simulink model "gm_ZynqBF_2tx_fpga"  (R2018b)
settings: Solver=FixedStepDiscrete  StartTime=0.0  StopTime=10.0  FixedStep=(1/420e3)/128  RelTol=1e-3
undefined symbols (not defined in the file or in its folder): a, b, c
libraries: hdlsllib x873, simulink x349
(part 40 of 40)

== matlab function gm_ZynqBF_2tx_fpga/channel_estimator/peakdetect_ch1/correlator1/rx_ram_q_instance17/get_bit/get_bit ==
  data: u input; y output; ind input
function y = fcn(u,ind)
%#codegen

y = logical(bitget(u,ind));

== matlab function gm_ZynqBF_2tx_fpga/channel_estimator/peakdetect_ch1/correlator1/rx_ram_q_instance18/get_bit/get_bit ==
  data: u input; y output; ind input
function y = fcn(u,ind)
%#codegen

y = logical(bitget(u,ind));

== matlab function gm_ZynqBF_2tx_fpga/channel_estimator/peakdetect_ch1/correlator1/rx_ram_q_instance19/get_bit/get_bit ==
  data: u input; y output; ind input
function y = fcn(u,ind)
%#codegen

y = logical(bitget(u,ind));

== matlab function gm_ZynqBF_2tx_fpga/channel_estimator/peakdetect_ch1/correlator1/rx_ram_q_instance20/get_bit/get_bit ==
  data: u input; y output; ind input
function y = fcn(u,ind)
%#codegen

y = logical(bitget(u,ind));

== matlab function gm_ZynqBF_2tx_fpga/channel_estimator/peakdetect_ch1/correlator1/rx_ram_q_instance21/get_bit/get_bit ==
  data: u input; y output; ind input
function y = fcn(u,ind)
%#codegen

y = logical(bitget(u,ind));

== matlab function gm_ZynqBF_2tx_fpga/channel_estimator/peakdetect_ch1/correlator1/rx_ram_q_instance22/get_bit/get_bit ==
  data: u input; y output; ind input
function y = fcn(u,ind)
%#codegen

y = logical(bitget(u,ind));

== matlab function gm_ZynqBF_2tx_fpga/channel_estimator/peakdetect_ch1/correlator1/rx_ram_q_instance23/get_bit/get_bit ==
  data: u input; y output; ind input
function y = fcn(u,ind)
%#codegen

y = logical(bitget(u,ind));

== matlab function gm_ZynqBF_2tx_fpga/channel_estimator/peakdetect_ch1/correlator1/rx_ram_q_instance24/get_bit/get_bit ==
  data: u input; y output; ind input
function y = fcn(u,ind)
%#codegen

y = logical(bitget(u,ind));

== matlab function gm_ZynqBF_2tx_fpga/channel_estimator/peakdetect_ch1/correlator1/rx_ram_q_instance25/get_bit/get_bit ==
  data: u input; y output; ind input
function y = fcn(u,ind)
%#codegen

y = logical(bitget(u,ind));

== matlab function gm_ZynqBF_2tx_fpga/channel_estimator/peakdetect_ch1/correlator1/rx_ram_q_instance26/get_bit/get_bit ==
  data: u input; y output; ind input
function y = fcn(u,ind)
%#codegen

y = logical(bitget(u,ind));

== matlab function gm_ZynqBF_2tx_fpga/channel_estimator/peakdetect_ch1/correlator1/rx_ram_q_instance27/get_bit/get_bit ==
  data: u input; y output; ind input
function y = fcn(u,ind)
%#codegen

y = logical(bitget(u,ind));

== matlab function gm_ZynqBF_2tx_fpga/channel_estimator/peakdetect_ch1/correlator1/rx_ram_q_instance28/get_bit/get_bit ==
  data: u input; y output; ind input
function y = fcn(u,ind)
%#codegen

y = logical(bitget(u,ind));

== matlab function gm_ZynqBF_2tx_fpga/channel_estimator/peakdetect_ch1/correlator1/rx_ram_q_instance29/get_bit/get_bit ==
  data: u input; y output; ind input
function y = fcn(u,ind)
%#codegen

y = logical(bitget(u,ind));

== matlab function gm_ZynqBF_2tx_fpga/channel_estimator/peakdetect_ch1/correlator1/rx_ram_q_instance30/get_bit/get_bit ==
  data: u input; y output; ind input
function y = fcn(u,ind)
%#codegen

y = logical(bitget(u,ind));

== matlab function gm_ZynqBF_2tx_fpga/channel_estimator/peakdetect_ch1/correlator1/rx_ram_q_instance31/get_bit/get_bit ==
  data: u input; y output; ind input
function y = fcn(u,ind)
%#codegen

y = logical(bitget(u,ind));

== matlab function gm_ZynqBF_2tx_fpga/channel_estimator/peakdetect_ch1/correlator1/rx_ram_q_instance32/get_bit/get_bit ==
  data: u input; y output; ind input
function y = fcn(u,ind)
%#codegen

y = logical(bitget(u,ind));

== matlab function gm_ZynqBF_2tx_fpga/channel_estimator/peakdetect_ch1/correlator1/rx_ram_q_instance33/get_bit/get_bit ==
  data: u input; y output; ind input
function y = fcn(u,ind)
%#codegen

y = logical(bitget(u,ind));

== matlab function gm_ZynqBF_2tx_fpga/channel_estimator/peakdetect_ch1/correlator1/rx_ram_q_instance34/get_bit/get_bit ==
  data: u input; y output; ind input
function y = fcn(u,ind)
%#codegen

y = logical(bitget(u,ind));

== matlab function gm_ZynqBF_2tx_fpga/channel_estimator/peakdetect_ch1/correlator1/rx_ram_q_instance35/get_bit/get_bit ==
  data: u input; y output; ind input
function y = fcn(u,ind)
%#codegen

y = logical(bitget(u,ind));

== matlab function gm_ZynqBF_2tx_fpga/channel_estimator/peakdetect_ch1/correlator1/rx_ram_q_instance36/get_bit/get_bit ==
  data: u input; y output; ind input
function y = fcn(u,ind)
%#codegen

y = logical(bitget(u,ind));

== matlab function gm_ZynqBF_2tx_fpga/channel_estimator/peakdetect_ch1/correlator1/rx_ram_q_instance37/get_bit/get_bit ==
  data: u input; y output; ind input
function y = fcn(u,ind)
%#codegen

y = logical(bitget(u,ind));

== matlab function gm_ZynqBF_2tx_fpga/channel_estimator/peakdetect_ch1/correlator1/rx_ram_q_instance38/get_bit/get_bit ==
  data: u input; y output; ind input
function y = fcn(u,ind)
%#codegen

y = logical(bitget(u,ind));

== matlab function gm_ZynqBF_2tx_fpga/channel_estimator/peakdetect_ch1/correlator1/rx_ram_q_instance39/get_bit/get_bit ==
  data: u input; y output; ind input
function y = fcn(u,ind)
%#codegen

y = logical(bitget(u,ind));

== matlab function gm_ZynqBF_2tx_fpga/channel_estimator/peakdetect_ch1/correlator1/rx_ram_q_instance40/get_bit/get_bit ==
  data: u input; y output; ind input
function y = fcn(u,ind)
%#codegen

y = logical(bitget(u,ind));

== matlab function gm_ZynqBF_2tx_fpga/channel_estimator/peakdetect_ch1/correlator1/rx_ram_q_instance41/get_bit/get_bit ==
  data: u input; y output; ind input
function y = fcn(u,ind)
%#codegen

y = logical(bitget(u,ind));

== matlab function gm_ZynqBF_2tx_fpga/channel_estimator/peakdetect_ch1/correlator1/rx_ram_q_instance42/get_bit/get_bit ==
  data: u input; y output; ind input
function y = fcn(u,ind)
%#codegen

y = logical(bitget(u,ind));

== matlab function gm_ZynqBF_2tx_fpga/channel_estimator/peakdetect_ch1/correlator1/rx_ram_q_instance43/get_bit/get_bit ==
  data: u input; y output; ind input
function y = fcn(u,ind)
%#codegen

y = logical(bitget(u,ind));

== matlab function gm_ZynqBF_2tx_fpga/channel_estimator/peakdetect_ch1/correlator1/rx_ram_q_instance44/get_bit/get_bit ==
  data: u input; y output; ind input
function y = fcn(u,ind)
%#codegen

y = logical(bitget(u,ind));

== matlab function gm_ZynqBF_2tx_fpga/channel_estimator/peakdetect_ch1/correlator1/rx_ram_q_instance45/get_bit/get_bit ==
  data: u input; y output; ind input
function y = fcn(u,ind)
%#codegen

y = logical(bitget(u,ind));

== matlab function gm_ZynqBF_2tx_fpga/channel_estimator/peakdetect_ch1/correlator1/rx_ram_q_instance46/get_bit/get_bit ==
  data: u input; y output; ind input
function y = fcn(u,ind)
%#codegen

y = logical(bitget(u,ind));

== matlab function gm_ZynqBF_2tx_fpga/channel_estimator/peakdetect_ch1/correlator1/rx_ram_q_instance47/get_bit/get_bit ==
  data: u input; y output; ind input
function y = fcn(u,ind)
%#codegen

y = logical(bitget(u,ind));

== matlab function gm_ZynqBF_2tx_fpga/channel_estimator/peakdetect_ch1/correlator1/rx_ram_q_instance48/get_bit/get_bit ==
  data: u input; y output; ind input
function y = fcn(u,ind)
%#codegen

y = logical(bitget(u,ind));

== matlab function gm_ZynqBF_2tx_fpga/channel_estimator/peakdetect_ch1/correlator1/rx_ram_q_instance49/get_bit/get_bit ==
  data: u input; y output; ind input
function y = fcn(u,ind)
%#codegen

y = logical(bitget(u,ind));

== matlab function gm_ZynqBF_2tx_fpga/channel_estimator/peakdetect_ch1/correlator1/rx_ram_q_instance50/get_bit/get_bit ==
  data: u input; y output; ind input
function y = fcn(u,ind)
%#codegen

y = logical(bitget(u,ind));

== matlab function gm_ZynqBF_2tx_fpga/channel_estimator/peakdetect_ch1/correlator1/rx_ram_q_instance51/get_bit/get_bit ==
  data: u input; y output; ind input
function y = fcn(u,ind)
%#codegen

y = logical(bitget(u,ind));

== matlab function gm_ZynqBF_2tx_fpga/channel_estimator/peakdetect_ch1/correlator1/rx_ram_q_instance52/get_bit/get_bit ==
  data: u input; y output; ind input
function y = fcn(u,ind)
%#codegen

y = logical(bitget(u,ind));

== matlab function gm_ZynqBF_2tx_fpga/channel_estimator/peakdetect_ch1/correlator1/rx_ram_q_instance53/get_bit/get_bit ==
  data: u input; y output; ind input
function y = fcn(u,ind)
%#codegen

y = logical(bitget(u,ind));

== matlab function gm_ZynqBF_2tx_fpga/channel_estimator/peakdetect_ch1/correlator1/rx_ram_q_instance54/get_bit/get_bit ==
  data: u input; y output; ind input
function y = fcn(u,ind)
%#codegen

y = logical(bitget(u,ind));

== matlab function gm_ZynqBF_2tx_fpga/channel_estimator/peakdetect_ch1/correlator1/rx_ram_q_instance55/get_bit/get_bit ==
  data: u input; y output; ind input
function y = fcn(u,ind)
%#codegen

y = logical(bitget(u,ind));

== matlab function gm_ZynqBF_2tx_fpga/channel_estimator/peakdetect_ch1/correlator1/rx_ram_q_instance56/get_bit/get_bit ==
  data: u input; y output; ind input
function y = fcn(u,ind)
%#codegen

y = logical(bitget(u,ind));

== matlab function gm_ZynqBF_2tx_fpga/channel_estimator/peakdetect_ch1/correlator1/rx_ram_q_instance57/get_bit/get_bit ==
  data: u input; y output; ind input
function y = fcn(u,ind)
%#codegen

y = logical(bitget(u,ind));

== matlab function gm_ZynqBF_2tx_fpga/channel_estimator/peakdetect_ch1/correlator1/rx_ram_q_instance58/get_bit/get_bit ==
  data: u input; y output; ind input
function y = fcn(u,ind)
%#codegen

y = logical(bitget(u,ind));

== matlab function gm_ZynqBF_2tx_fpga/channel_estimator/peakdetect_ch1/correlator1/rx_ram_q_instance59/get_bit/get_bit ==
  data: u input; y output; ind input
function y = fcn(u,ind)
%#codegen

y = logical(bitget(u,ind));

== matlab function gm_ZynqBF_2tx_fpga/channel_estimator/peakdetect_ch1/correlator1/rx_ram_q_instance60/get_bit/get_bit ==
  data: u input; y output; ind input
function y = fcn(u,ind)
%#codegen

y = logical(bitget(u,ind));

== matlab function gm_ZynqBF_2tx_fpga/channel_estimator/peakdetect_ch1/correlator1/rx_ram_q_instance61/get_bit/get_bit ==
  data: u input; y output; ind input
function y = fcn(u,ind)
%#codegen

y = logical(bitget(u,ind));

== matlab function gm_ZynqBF_2tx_fpga/channel_estimator/peakdetect_ch1/correlator1/rx_ram_q_instance62/get_bit/get_bit ==
  data: u input; y output; ind input
function y = fcn(u,ind)
%#codegen

y = logical(bitget(u,ind));

== matlab function gm_ZynqBF_2tx_fpga/channel_estimator/peakdetect_ch1/correlator1/rx_ram_q_instance63/get_bit/get_bit ==
  data: u input; y output; ind input
function y = fcn(u,ind)
%#codegen

y = logical(bitget(u,ind));

== matlab function gm_ZynqBF_2tx_fpga/channel_estimator/peakdetect_ch1/correlator1/rx_ram_q_instance64/get_bit/get_bit ==
  data: u input; y output; ind input
function y = fcn(u,ind)
%#codegen

y = logical(bitget(u,ind));

== matlab function gm_ZynqBF_2tx_fpga/channel_estimator/ram_rd_counter/select_inputs/select_inputs ==
  data: en1 input; y output; en2 input; in1 input; in2 input
function y = fcn(en1, en2, in1, in2)
%#codegen

if (en1 && en2)
    y = zeros(1,1,'like',in1);
elseif (en1)
    y = in1;
elseif (en2)
    y = in2;
else
    y = zeros(1,1,'like',in1);
end

== matlab function gm_ZynqBF_2tx_fpga/channel_estimator/peakdetect_ch2/correlator2/rx_ram_i_instance1/get_bit/get_bit ==
  data: u input; y output; ind input
function y = fcn(u,ind)
%#codegen

y = logical(bitget(u,ind));

== matlab function gm_ZynqBF_2tx_fpga/channel_estimator/peakdetect_ch2/correlator2/rx_ram_q_instance1/get_bit/get_bit ==
  data: u input; y output; ind input
function y = fcn(u,ind)
%#codegen

y = logical(bitget(u,ind));

== matlab function gm_ZynqBF_2tx_fpga/channel_estimator/peakdetect_ch2/correlator2/all_u/all_u ==
  data: u input size=8; y output size=1
function y = fcn(u)

y = all(u);

== matlab function gm_ZynqBF_2tx_fpga/channel_estimator/peakdetect_ch2/correlator2/all_u1/all_u ==
  data: u input size=8; y output size=1
function y = fcn(u)

y = all(u);

== matlab function gm_ZynqBF_2tx_fpga/channel_estimator/peakdetect_ch2/correlator2/shift_rx/shift_rx ==
  data: u input; y output size=64; shift input [1..64]
function y = fcn(u, shift)
%#codegen
% y = zeros(64,1,'like',u);
y = circshift(u,-(int8(shift)));

== matlab function gm_ZynqBF_2tx_fpga/channel_estimator/peakdetect_ch2/correlator2/shift_rx1/shift_rx ==
  data: u input; y output size=64; shift input [1..64]
function y = fcn(u, shift)
%#codegen
% y = zeros(64,1,'like',u);
y = circshift(u,-(int8(shift)));

== matlab function gm_ZynqBF_2tx_fpga/channel_estimator/peakdetect_ch2/correlator2/rx_ram_i_instance2/get_bit/get_bit ==
  data: u input; y output; ind input
function y = fcn(u,ind)
%#codegen

y = logical(bitget(u,ind));

== matlab function gm_ZynqBF_2tx_fpga/channel_estimator/peakdetect_ch2/correlator2/rx_ram_i_instance3/get_bit/get_bit ==
  data: u input; y output; ind input
function y = fcn(u,ind)
%#codegen

y = logical(bitget(u,ind));

== matlab function gm_ZynqBF_2tx_fpga/channel_estimator/peakdetect_ch2/correlator2/rx_ram_i_instance4/get_bit/get_bit ==
  data: u input; y output; ind input
function y = fcn(u,ind)
%#codegen

y = logical(bitget(u,ind));

== matlab function gm_ZynqBF_2tx_fpga/channel_estimator/peakdetect_ch2/correlator2/rx_ram_i_instance5/get_bit/get_bit ==
  data: u input; y output; ind input
function y = fcn(u,ind)
%#codegen

y = logical(bitget(u,ind));

== matlab function gm_ZynqBF_2tx_fpga/channel_estimator/peakdetect_ch2/correlator2/rx_ram_i_instance6/get_bit/get_bit ==
  data: u input; y output; ind input
function y = fcn(u,ind)
%#codegen

y = logical(bitget(u,ind));

== matlab function gm_ZynqBF_2tx_fpga/channel_estimator/peakdetect_ch2/correlator2/rx_ram_i_instance7/get_bit/get_bit ==
  data: u input; y output; ind input
function y = fcn(u,ind)
%#codegen

y = logical(bitget(u,ind));

== matlab function gm_ZynqBF_2tx_fpga/channel_estimator/peakdetect_ch2/correlator2/rx_ram_i_instance8/get_bit/get_bit ==
  data: u input; y output; ind input
function y = fcn(u,ind)
%#codegen

y = logical(bitget(u,ind));

== matlab function gm_ZynqBF_2tx_fpga/channel_estimator/peakdetect_ch2/correlator2/rx_ram_i_instance9/get_bit/get_bit ==
  data: u input; y output; ind input
function y = fcn(u,ind)
%#codegen

y = logical(bitget(u,ind));

== matlab function gm_ZynqBF_2tx_fpga/channel_estimator/peakdetect_ch2/correlator2/rx_ram_i_instance10/get_bit/get_bit ==
  data: u input; y output; ind input
function y = fcn(u,ind)
%#codegen

y = logical(bitget(u,ind));

== matlab function gm_ZynqBF_2tx_fpga/channel_estimator/peakdetect_ch2/correlator2/rx_ram_i_instance11/get_bit/get_bit ==
  data: u input; y output; ind input
function y = fcn(u,ind)
%#codegen

y = logical(bitget(u,ind));

== matlab function gm_ZynqBF_2tx_fpga/channel_estimator/peakdetect_ch2/correlator2/rx_ram_i_instance12/get_bit/get_bit ==
  data: u input; y output; ind input
function y = fcn(u,ind)
%#codegen

y = logical(bitget(u,ind));

== matlab function gm_ZynqBF_2tx_fpga/channel_estimator/peakdetect_ch2/correlator2/rx_ram_i_instance13/get_bit/get_bit ==
  data: u input; y output; ind input
function y = fcn(u,ind)
%#codegen

y = logical(bitget(u,ind));

== matlab function gm_ZynqBF_2tx_fpga/channel_estimator/peakdetect_ch2/correlator2/rx_ram_i_instance14/get_bit/get_bit ==
  data: u input; y output; ind input
function y = fcn(u,ind)
%#codegen

y = logical(bitget(u,ind));

== matlab function gm_ZynqBF_2tx_fpga/channel_estimator/peakdetect_ch2/correlator2/rx_ram_i_instance15/get_bit/get_bit ==
  data: u input; y output; ind input
function y = fcn(u,ind)
%#codegen

y = logical(bitget(u,ind));

== matlab function gm_ZynqBF_2tx_fpga/channel_estimator/peakdetect_ch2/correlator2/rx_ram_i_instance16/get_bit/get_bit ==
  data: u input; y output; ind input
function y = fcn(u,ind)
%#codegen

y = logical(bitget(u,ind));

== matlab function gm_ZynqBF_2tx_fpga/channel_estimator/peakdetect_ch2/correlator2/rx_ram_i_instance17/get_bit/get_bit ==
  data: u input; y output; ind input
function y = fcn(u,ind)
%#codegen

y = logical(bitget(u,ind));

== matlab function gm_ZynqBF_2tx_fpga/channel_estimator/peakdetect_ch2/correlator2/rx_ram_i_instance18/get_bit/get_bit ==
  data: u input; y output; ind input
function y = fcn(u,ind)
%#codegen

y = logical(bitget(u,ind));

== matlab function gm_ZynqBF_2tx_fpga/channel_estimator/peakdetect_ch2/correlator2/rx_ram_i_instance19/get_bit/get_bit ==
  data: u input; y output; ind input
function y = fcn(u,ind)
%#codegen

y = logical(bitget(u,ind));

== matlab function gm_ZynqBF_2tx_fpga/channel_estimator/peakdetect_ch2/correlator2/rx_ram_i_instance20/get_bit/get_bit ==
  data: u input; y output; ind input
function y = fcn(u,ind)
%#codegen

y = logical(bitget(u,ind));

== matlab function gm_ZynqBF_2tx_fpga/channel_estimator/peakdetect_ch2/correlator2/rx_ram_i_instance21/get_bit/get_bit ==
  data: u input; y output; ind input
function y = fcn(u,ind)
%#codegen

y = logical(bitget(u,ind));

== matlab function gm_ZynqBF_2tx_fpga/channel_estimator/peakdetect_ch2/correlator2/rx_ram_i_instance22/get_bit/get_bit ==
  data: u input; y output; ind input
function y = fcn(u,ind)
%#codegen

y = logical(bitget(u,ind));

== matlab function gm_ZynqBF_2tx_fpga/channel_estimator/peakdetect_ch2/correlator2/rx_ram_i_instance23/get_bit/get_bit ==
  data: u input; y output; ind input
function y = fcn(u,ind)
%#codegen

y = logical(bitget(u,ind));

== matlab function gm_ZynqBF_2tx_fpga/channel_estimator/peakdetect_ch2/correlator2/rx_ram_i_instance24/get_bit/get_bit ==
  data: u input; y output; ind input
function y = fcn(u,ind)
%#codegen

y = logical(bitget(u,ind));

== matlab function gm_ZynqBF_2tx_fpga/channel_estimator/peakdetect_ch2/correlator2/rx_ram_i_instance25/get_bit/get_bit ==
  data: u input; y output; ind input
function y = fcn(u,ind)
%#codegen

y = logical(bitget(u,ind));

== matlab function gm_ZynqBF_2tx_fpga/channel_estimator/peakdetect_ch2/correlator2/rx_ram_i_instance26/get_bit/get_bit ==
  data: u input; y output; ind input
function y = fcn(u,ind)
%#codegen

y = logical(bitget(u,ind));

== matlab function gm_ZynqBF_2tx_fpga/channel_estimator/peakdetect_ch2/correlator2/rx_ram_i_instance27/get_bit/get_bit ==
  data: u input; y output; ind input
function y = fcn(u,ind)
%#codegen

y = logical(bitget(u,ind));

== matlab function gm_ZynqBF_2tx_fpga/channel_estimator/peakdetect_ch2/correlator2/rx_ram_i_instance28/get_bit/get_bit ==
  data: u input; y output; ind input
function y = fcn(u,ind)
%#codegen

y = logical(bitget(u,ind));

== matlab function gm_ZynqBF_2tx_fpga/channel_estimator/peakdetect_ch2/correlator2/rx_ram_i_instance29/get_bit/get_bit ==
  data: u input; y output; ind input
function y = fcn(u,ind)
%#codegen

y = logical(bitget(u,ind));

== matlab function gm_ZynqBF_2tx_fpga/channel_estimator/peakdetect_ch2/correlator2/rx_ram_i_instance30/get_bit/get_bit ==
  data: u input; y output; ind input
function y = fcn(u,ind)
%#codegen

y = logical(bitget(u,ind));

== matlab function gm_ZynqBF_2tx_fpga/channel_estimator/peakdetect_ch2/correlator2/rx_ram_i_instance31/get_bit/get_bit ==
  data: u input; y output; ind input
function y = fcn(u,ind)
%#codegen

y = logical(bitget(u,ind));

== matlab function gm_ZynqBF_2tx_fpga/channel_estimator/peakdetect_ch2/correlator2/rx_ram_i_instance32/get_bit/get_bit ==
  data: u input; y output; ind input
function y = fcn(u,ind)
%#codegen

y = logical(bitget(u,ind));

== matlab function gm_ZynqBF_2tx_fpga/channel_estimator/peakdetect_ch2/correlator2/rx_ram_i_instance33/get_bit/get_bit ==
  data: u input; y output; ind input
function y = fcn(u,ind)
%#codegen

y = logical(bitget(u,ind));

== matlab function gm_ZynqBF_2tx_fpga/channel_estimator/peakdetect_ch2/correlator2/rx_ram_i_instance34/get_bit/get_bit ==
  data: u input; y output; ind input
function y = fcn(u,ind)
%#codegen

y = logical(bitget(u,ind));

== matlab function gm_ZynqBF_2tx_fpga/channel_estimator/peakdetect_ch2/correlator2/rx_ram_i_instance35/get_bit/get_bit ==
  data: u input; y output; ind input
function y = fcn(u,ind)
%#codegen

y = logical(bitget(u,ind));

== matlab function gm_ZynqBF_2tx_fpga/channel_estimator/peakdetect_ch2/correlator2/rx_ram_i_instance36/get_bit/get_bit ==
  data: u input; y output; ind input
function y = fcn(u,ind)
%#codegen

y = logical(bitget(u,ind));

== matlab function gm_ZynqBF_2tx_fpga/channel_estimator/peakdetect_ch2/correlator2/rx_ram_i_instance37/get_bit/get_bit ==
  data: u input; y output; ind input
function y = fcn(u,ind)
%#codegen

y = logical(bitget(u,ind));

== matlab function gm_ZynqBF_2tx_fpga/channel_estimator/peakdetect_ch2/correlator2/rx_ram_i_instance38/get_bit/get_bit ==
  data: u input; y output; ind input
function y = fcn(u,ind)
%#codegen

y = logical(bitget(u,ind));

== matlab function gm_ZynqBF_2tx_fpga/channel_estimator/peakdetect_ch2/correlator2/rx_ram_i_instance39/get_bit/get_bit ==
  data: u input; y output; ind input
function y = fcn(u,ind)
%#codegen

y = logical(bitget(u,ind));

== matlab function gm_ZynqBF_2tx_fpga/channel_estimator/peakdetect_ch2/correlator2/rx_ram_i_instance40/get_bit/get_bit ==
  data: u input; y output; ind input
function y = fcn(u,ind)
%#codegen

y = logical(bitget(u,ind));

== matlab function gm_ZynqBF_2tx_fpga/channel_estimator/peakdetect_ch2/correlator2/rx_ram_i_instance41/get_bit/get_bit ==
  data: u input; y output; ind input
function y = fcn(u,ind)
%#codegen

y = logical(bitget(u,ind));

== matlab function gm_ZynqBF_2tx_fpga/channel_estimator/peakdetect_ch2/correlator2/rx_ram_i_instance42/get_bit/get_bit ==
  data: u input; y output; ind input
function y = fcn(u,ind)
%#codegen

y = logical(bitget(u,ind));

== matlab function gm_ZynqBF_2tx_fpga/channel_estimator/peakdetect_ch2/correlator2/rx_ram_i_instance43/get_bit/get_bit ==
  data: u input; y output; ind input
function y = fcn(u,ind)
%#codegen

y = logical(bitget(u,ind));

== matlab function gm_ZynqBF_2tx_fpga/channel_estimator/peakdetect_ch2/correlator2/rx_ram_i_instance44/get_bit/get_bit ==
  data: u input; y output; ind input
function y = fcn(u,ind)
%#codegen

y = logical(bitget(u,ind));

== matlab function gm_ZynqBF_2tx_fpga/channel_estimator/peakdetect_ch2/correlator2/rx_ram_i_instance45/get_bit/get_bit ==
  data: u input; y output; ind input
function y = fcn(u,ind)
%#codegen

y = logical(bitget(u,ind));

== matlab function gm_ZynqBF_2tx_fpga/channel_estimator/peakdetect_ch2/correlator2/rx_ram_i_instance46/get_bit/get_bit ==
  data: u input; y output; ind input
function y = fcn(u,ind)
%#codegen

y = logical(bitget(u,ind));

== matlab function gm_ZynqBF_2tx_fpga/channel_estimator/peakdetect_ch2/correlator2/rx_ram_i_instance47/get_bit/get_bit ==
  data: u input; y output; ind input
function y = fcn(u,ind)
%#codegen

y = logical(bitget(u,ind));

== matlab function gm_ZynqBF_2tx_fpga/channel_estimator/peakdetect_ch2/correlator2/rx_ram_i_instance48/get_bit/get_bit ==
  data: u input; y output; ind input
function y = fcn(u,ind)
%#codegen

y = logical(bitget(u,ind));

== matlab function gm_ZynqBF_2tx_fpga/channel_estimator/peakdetect_ch2/correlator2/rx_ram_i_instance49/get_bit/get_bit ==
  data: u input; y output; ind input
function y = fcn(u,ind)
%#codegen

y = logical(bitget(u,ind));

== matlab function gm_ZynqBF_2tx_fpga/channel_estimator/peakdetect_ch2/correlator2/rx_ram_i_instance50/get_bit/get_bit ==
  data: u input; y output; ind input
function y = fcn(u,ind)
%#codegen

y = logical(bitget(u,ind));

== matlab function gm_ZynqBF_2tx_fpga/channel_estimator/peakdetect_ch2/correlator2/rx_ram_i_instance51/get_bit/get_bit ==
  data: u input; y output; ind input
function y = fcn(u,ind)
%#codegen

y = logical(bitget(u,ind));

== matlab function gm_ZynqBF_2tx_fpga/channel_estimator/peakdetect_ch2/correlator2/rx_ram_i_instance52/get_bit/get_bit ==
  data: u input; y output; ind input
function y = fcn(u,ind)
%#codegen

y = logical(bitget(u,ind));

== matlab function gm_ZynqBF_2tx_fpga/channel_estimator/peakdetect_ch2/correlator2/rx_ram_i_instance53/get_bit/get_bit ==
  data: u input; y output; ind input
function y = fcn(u,ind)
%#codegen

y = logical(bitget(u,ind));

== matlab function gm_ZynqBF_2tx_fpga/channel_estimator/peakdetect_ch2/correlator2/rx_ram_i_instance54/get_bit/get_bit ==
  data: u input; y output; ind input
function y = fcn(u,ind)
%#codegen

y = logical(bitget(u,ind));

== matlab function gm_ZynqBF_2tx_fpga/channel_estimator/peakdetect_ch2/correlator2/rx_ram_i_instance55/get_bit/get_bit ==
  data: u input; y output; ind input
function y = fcn(u,ind)
%#codegen

y = logical(bitget(u,ind));

== matlab function gm_ZynqBF_2tx_fpga/channel_estimator/peakdetect_ch2/correlator2/rx_ram_i_instance56/get_bit/get_bit ==
  data: u input; y output; ind input
function y = fcn(u,ind)
%#codegen

y = logical(bitget(u,ind));

== matlab function gm_ZynqBF_2tx_fpga/channel_estimator/peakdetect_ch2/correlator2/rx_ram_i_instance57/get_bit/get_bit ==
  data: u input; y output; ind input
function y = fcn(u,ind)
%#codegen

y = logical(bitget(u,ind));

== matlab function gm_ZynqBF_2tx_fpga/channel_estimator/peakdetect_ch2/correlator2/rx_ram_i_instance58/get_bit/get_bit ==
  data: u input; y output; ind input
function y = fcn(u,ind)
%#codegen

y = logical(bitget(u,ind));

== matlab function gm_ZynqBF_2tx_fpga/channel_estimator/peakdetect_ch2/correlator2/rx_ram_i_instance59/get_bit/get_bit ==
  data: u input; y output; ind input
function y = fcn(u,ind)
%#codegen

y = logical(bitget(u,ind));

== matlab function gm_ZynqBF_2tx_fpga/channel_estimator/peakdetect_ch2/correlator2/rx_ram_i_instance60/get_bit/get_bit ==
  data: u input; y output; ind input
function y = fcn(u,ind)
%#codegen

y = logical(bitget(u,ind));

== matlab function gm_ZynqBF_2tx_fpga/channel_estimator/peakdetect_ch2/correlator2/rx_ram_i_instance61/get_bit/get_bit ==
  data: u input; y output; ind input
function y = fcn(u,ind)
%#codegen

y = logical(bitget(u,ind));

== matlab function gm_ZynqBF_2tx_fpga/channel_estimator/peakdetect_ch2/correlator2/rx_ram_i_instance62/get_bit/get_bit ==
  data: u input; y output; ind input
function y = fcn(u,ind)
%#codegen

y = logical(bitget(u,ind));

== matlab function gm_ZynqBF_2tx_fpga/channel_estimator/peakdetect_ch2/correlator2/rx_ram_i_instance63/get_bit/get_bit ==
  data: u input; y output; ind input
function y = fcn(u,ind)
%#codegen

y = logical(bitget(u,ind));

== matlab function gm_ZynqBF_2tx_fpga/channel_estimator/peakdetect_ch2/correlator2/rx_ram_i_instance64/get_bit/get_bit ==
  data: u input; y output; ind input
function y = fcn(u,ind)
%#codegen

y = logical(bitget(u,ind));

== matlab function gm_ZynqBF_2tx_fpga/channel_estimator/peakdetect_ch2/correlator2/rx_ram_q_instance2/get_bit/get_bit ==
  data: u input; y output; ind input
function y = fcn(u,ind)
%#codegen

y = logical(bitget(u,ind));

== matlab function gm_ZynqBF_2tx_fpga/channel_estimator/peakdetect_ch2/correlator2/rx_ram_q_instance3/get_bit/get_bit ==
  data: u input; y output; ind input
function y = fcn(u,ind)
%#codegen

y = logical(bitget(u,ind));

== matlab function gm_ZynqBF_2tx_fpga/channel_estimator/peakdetect_ch2/correlator2/rx_ram_q_instance4/get_bit/get_bit ==
  data: u input; y output; ind input
function y = fcn(u,ind)
%#codegen

y = logical(bitget(u,ind));

== matlab function gm_ZynqBF_2tx_fpga/channel_estimator/peakdetect_ch2/correlator2/rx_ram_q_instance5/get_bit/get_bit ==
  data: u input; y output; ind input
function y = fcn(u,ind)
%#codegen

y = logical(bitget(u,ind));

== matlab function gm_ZynqBF_2tx_fpga/channel_estimator/peakdetect_ch2/correlator2/rx_ram_q_instance6/get_bit/get_bit ==
  data: u input; y output; ind input
function y = fcn(u,ind)
%#codegen

y = logical(bitget(u,ind));

== matlab function gm_ZynqBF_2tx_fpga/channel_estimator/peakdetect_ch2/correlator2/rx_ram_q_instance7/get_bit/get_bit ==
  data: u input; y output; ind input
function y = fcn(u,ind)
%#codegen

y = logical(bitget(u,ind));

== matlab function gm_ZynqBF_2tx_fpga/channel_estimator/peakdetect_ch2/correlator2/rx_ram_q_instance8/get_bit/get_bit ==
  data: u input; y output; ind input
function y = fcn(u,ind)
%#codegen

y = logical(bitget(u,ind));

== matlab function gm_ZynqBF_2tx_fpga/channel_estimator/peakdetect_ch2/correlator2/rx_ram_q_instance9/get_bit/get_bit ==
  data: u input; y output; ind input
function y = fcn(u,ind)
%#codegen

y = logical(bitget(u,ind));

== matlab function gm_ZynqBF_2tx_fpga/channel_estimator/peakdetect_ch2/correlator2/rx_ram_q_instance10/get_bit/get_bit ==
  data: u input; y output; ind input
function y = fcn(u,ind)
%#codegen

y = logical(bitget(u,ind));

== matlab function gm_ZynqBF_2tx_fpga/channel_estimator/peakdetect_ch2/correlator2/rx_ram_q_instance11/get_bit/get_bit ==
  data: u input; y output; ind input
function y = fcn(u,ind)
%#codegen

y = logical(bitget(u,ind));

== matlab function gm_ZynqBF_2tx_fpga/channel_estimator/peakdetect_ch2/correlator2/rx_ram_q_instance12/get_bit/get_bit ==
  data: u input; y output; ind input
function y = fcn(u,ind)
%#codegen

y = logical(bitget(u,ind));

== matlab function gm_ZynqBF_2tx_fpga/channel_estimator/peakdetect_ch2/correlator2/rx_ram_q_instance13/get_bit/get_bit ==
  data: u input; y output; ind input
function y = fcn(u,ind)
%#codegen

y = logical(bitget(u,ind));

== matlab function gm_ZynqBF_2tx_fpga/channel_estimator/peakdetect_ch2/correlator2/rx_ram_q_instance14/get_bit/get_bit ==
  data: u input; y output; ind input
function y = fcn(u,ind)
%#codegen

y = logical(bitget(u,ind));

== matlab function gm_ZynqBF_2tx_fpga/channel_estimator/peakdetect_ch2/correlator2/rx_ram_q_instance15/get_bit/get_bit ==
  data: u input; y output; ind input
function y = fcn(u,ind)
%#codegen

y = logical(bitget(u,ind));

== matlab function gm_ZynqBF_2tx_fpga/channel_estimator/peakdetect_ch2/correlator2/rx_ram_q_instance16/get_bit/get_bit ==
  data: u input; y output; ind input
function y = fcn(u,ind)
%#codegen

y = logical(bitget(u,ind));

== matlab function gm_ZynqBF_2tx_fpga/channel_estimator/peakdetect_ch2/correlator2/rx_ram_q_instance17/get_bit/get_bit ==
  data: u input; y output; ind input
function y = fcn(u,ind)
%#codegen

y = logical(bitget(u,ind));

== matlab function gm_ZynqBF_2tx_fpga/channel_estimator/peakdetect_ch2/correlator2/rx_ram_q_instance18/get_bit/get_bit ==
  data: u input; y output; ind input
function y = fcn(u,ind)
%#codegen

y = logical(bitget(u,ind));

== matlab function gm_ZynqBF_2tx_fpga/channel_estimator/peakdetect_ch2/correlator2/rx_ram_q_instance19/get_bit/get_bit ==
  data: u input; y output; ind input
function y = fcn(u,ind)
%#codegen

y = logical(bitget(u,ind));

== matlab function gm_ZynqBF_2tx_fpga/channel_estimator/peakdetect_ch2/correlator2/rx_ram_q_instance20/get_bit/get_bit ==
  data: u input; y output; ind input
function y = fcn(u,ind)
%#codegen

y = logical(bitget(u,ind));

== matlab function gm_ZynqBF_2tx_fpga/channel_estimator/peakdetect_ch2/correlator2/rx_ram_q_instance21/get_bit/get_bit ==
  data: u input; y output; ind input
function y = fcn(u,ind)
%#codegen

y = logical(bitget(u,ind));

== matlab function gm_ZynqBF_2tx_fpga/channel_estimator/peakdetect_ch2/correlator2/rx_ram_q_instance22/get_bit/get_bit ==
  data: u input; y output; ind input
function y = fcn(u,ind)
%#codegen

y = logical(bitget(u,ind));

== matlab function gm_ZynqBF_2tx_fpga/channel_estimator/peakdetect_ch2/correlator2/rx_ram_q_instance23/get_bit/get_bit ==
  data: u input; y output; ind input
function y = fcn(u,ind)
%#codegen

y = logical(bitget(u,ind));

== matlab function gm_ZynqBF_2tx_fpga/channel_estimator/peakdetect_ch2/correlator2/rx_ram_q_instance24/get_bit/get_bit ==
  data: u input; y output; ind input
function y = fcn(u,ind)
%#codegen

y = logical(bitget(u,ind));

== matlab function gm_ZynqBF_2tx_fpga/channel_estimator/peakdetect_ch2/correlator2/rx_ram_q_instance25/get_bit/get_bit ==
  data: u input; y output; ind input
function y = fcn(u,ind)
%#codegen

y = logical(bitget(u,ind));

== matlab function gm_ZynqBF_2tx_fpga/channel_estimator/peakdetect_ch2/correlator2/rx_ram_q_instance26/get_bit/get_bit ==
  data: u input; y output; ind input
function y = fcn(u,ind)
%#codegen

y = logical(bitget(u,ind));

== matlab function gm_ZynqBF_2tx_fpga/channel_estimator/peakdetect_ch2/correlator2/rx_ram_q_instance27/get_bit/get_bit ==
  data: u input; y output; ind input
function y = fcn(u,ind)
%#codegen

y = logical(bitget(u,ind));

== matlab function gm_ZynqBF_2tx_fpga/channel_estimator/peakdetect_ch2/correlator2/rx_ram_q_instance28/get_bit/get_bit ==
  data: u input; y output; ind input
function y = fcn(u,ind)
%#codegen

y = logical(bitget(u,ind));

== matlab function gm_ZynqBF_2tx_fpga/channel_estimator/peakdetect_ch2/correlator2/rx_ram_q_instance29/get_bit/get_bit ==
  data: u input; y output; ind input
function y = fcn(u,ind)
%#codegen

y = logical(bitget(u,ind));

== matlab function gm_ZynqBF_2tx_fpga/channel_estimator/peakdetect_ch2/correlator2/rx_ram_q_instance30/get_bit/get_bit ==
  data: u input; y output; ind input
function y = fcn(u,ind)
%#codegen

y = logical(bitget(u,ind));

== matlab function gm_ZynqBF_2tx_fpga/channel_estimator/peakdetect_ch2/correlator2/rx_ram_q_instance31/get_bit/get_bit ==
  data: u input; y output; ind input
function y = fcn(u,ind)
%#codegen

y = logical(bitget(u,ind));

== matlab function gm_ZynqBF_2tx_fpga/channel_estimator/peakdetect_ch2/correlator2/rx_ram_q_instance32/get_bit/get_bit ==
  data: u input; y output; ind input
function y = fcn(u,ind)
%#codegen

y = logical(bitget(u,ind));

== matlab function gm_ZynqBF_2tx_fpga/channel_estimator/peakdetect_ch2/correlator2/rx_ram_q_instance33/get_bit/get_bit ==
  data: u input; y output; ind input
function y = fcn(u,ind)
%#codegen

y = logical(bitget(u,ind));

== matlab function gm_ZynqBF_2tx_fpga/channel_estimator/peakdetect_ch2/correlator2/rx_ram_q_instance34/get_bit/get_bit ==
  data: u input; y output; ind input
function y = fcn(u,ind)
%#codegen

y = logical(bitget(u,ind));

== matlab function gm_ZynqBF_2tx_fpga/channel_estimator/peakdetect_ch2/correlator2/rx_ram_q_instance35/get_bit/get_bit ==
  data: u input; y output; ind input
function y = fcn(u,ind)
%#codegen

y = logical(bitget(u,ind));

== matlab function gm_ZynqBF_2tx_fpga/channel_estimator/peakdetect_ch2/correlator2/rx_ram_q_instance36/get_bit/get_bit ==
  data: u input; y output; ind input
function y = fcn(u,ind)
%#codegen

y = logical(bitget(u,ind));

== matlab function gm_ZynqBF_2tx_fpga/channel_estimator/peakdetect_ch2/correlator2/rx_ram_q_instance37/get_bit/get_bit ==
  data: u input; y output; ind input
function y = fcn(u,ind)
%#codegen

y = logical(bitget(u,ind));

== matlab function gm_ZynqBF_2tx_fpga/channel_estimator/peakdetect_ch2/correlator2/rx_ram_q_instance38/get_bit/get_bit ==
  data: u input; y output; ind input
function y = fcn(u,ind)
%#codegen

y = logical(bitget(u,ind));

== matlab function gm_ZynqBF_2tx_fpga/channel_estimator/peakdetect_ch2/correlator2/rx_ram_q_instance39/get_bit/get_bit ==
  data: u input; y output; ind input
function y = fcn(u,ind)
%#codegen

y = logical(bitget(u,ind));

== matlab function gm_ZynqBF_2tx_fpga/channel_estimator/peakdetect_ch2/correlator2/rx_ram_q_instance40/get_bit/get_bit ==
  data: u input; y output; ind input
function y = fcn(u,ind)
%#codegen

y = logical(bitget(u,ind));

== matlab function gm_ZynqBF_2tx_fpga/channel_estimator/peakdetect_ch2/correlator2/rx_ram_q_instance41/get_bit/get_bit ==
  data: u input; y output; ind input
function y = fcn(u,ind)
%#codegen

y = logical(bitget(u,ind));

== matlab function gm_ZynqBF_2tx_fpga/channel_estimator/peakdetect_ch2/correlator2/rx_ram_q_instance42/get_bit/get_bit ==
  data: u input; y output; ind input
function y = fcn(u,ind)
%#codegen

y = logical(bitget(u,ind));

== matlab function gm_ZynqBF_2tx_fpga/channel_estimator/peakdetect_ch2/correlator2/rx_ram_q_instance43/get_bit/get_bit ==
  data: u input; y output; ind input
function y = fcn(u,ind)
%#codegen

y = logical(bitget(u,ind));

== matlab function gm_ZynqBF_2tx_fpga/channel_estimator/peakdetect_ch2/correlator2/rx_ram_q_instance44/get_bit/get_bit ==
  data: u input; y output; ind input
function y = fcn(u,ind)
%#codegen

y = logical(bitget(u,ind));

== matlab function gm_ZynqBF_2tx_fpga/channel_estimator/peakdetect_ch2/correlator2/rx_ram_q_instance45/get_bit/get_bit ==
  data: u input; y output; ind input
function y = fcn(u,ind)
%#codegen

y = logical(bitget(u,ind));

== matlab function gm_ZynqBF_2tx_fpga/channel_estimator/peakdetect_ch2/correlator2/rx_ram_q_instance46/get_bit/get_bit ==
  data: u input; y output; ind input
function y = fcn(u,ind)
%#codegen

y = logical(bitget(u,ind));

== matlab function gm_ZynqBF_2tx_fpga/channel_estimator/peakdetect_ch2/correlator2/rx_ram_q_instance47/get_bit/get_bit ==
  data: u input; y output; ind input
function y = fcn(u,ind)
%#codegen

y = logical(bitget(u,ind));

== matlab function gm_ZynqBF_2tx_fpga/channel_estimator/peakdetect_ch2/correlator2/rx_ram_q_instance48/get_bit/get_bit ==
  data: u input; y output; ind input
function y = fcn(u,ind)
%#codegen

y = logical(bitget(u,ind));

== matlab function gm_ZynqBF_2tx_fpga/channel_estimator/peakdetect_ch2/correlator2/rx_ram_q_instance49/get_bit/get_bit ==
  data: u input; y output; ind input
function y = fcn(u,ind)
%#codegen

y = logical(bitget(u,ind));

== matlab function gm_ZynqBF_2tx_fpga/channel_estimator/peakdetect_ch2/correlator2/rx_ram_q_instance50/get_bit/get_bit ==
  data: u input; y output; ind input
function y = fcn(u,ind)
%#codegen

y = logical(bitget(u,ind));

== matlab function gm_ZynqBF_2tx_fpga/channel_estimator/peakdetect_ch2/correlator2/rx_ram_q_instance51/get_bit/get_bit ==
  data: u input; y output; ind input
function y = fcn(u,ind)
%#codegen

y = logical(bitget(u,ind));

== matlab function gm_ZynqBF_2tx_fpga/channel_estimator/peakdetect_ch2/correlator2/rx_ram_q_instance52/get_bit/get_bit ==
  data: u input; y output; ind input
function y = fcn(u,ind)
%#codegen

y = logical(bitget(u,ind));

== matlab function gm_ZynqBF_2tx_fpga/channel_estimator/peakdetect_ch2/correlator2/rx_ram_q_instance53/get_bit/get_bit ==
  data: u input; y output; ind input
function y = fcn(u,ind)
%#codegen

y = logical(bitget(u,ind));

== matlab function gm_ZynqBF_2tx_fpga/channel_estimator/peakdetect_ch2/correlator2/rx_ram_q_instance54/get_bit/get_bit ==
  data: u input; y output; ind input
function y = fcn(u,ind)
%#codegen

y = logical(bitget(u,ind));

== matlab function gm_ZynqBF_2tx_fpga/channel_estimator/peakdetect_ch2/correlator2/rx_ram_q_instance55/get_bit/get_bit ==
  data: u input; y output; ind input
function y = fcn(u,ind)
%#codegen

y = logical(bitget(u,ind));

== matlab function gm_ZynqBF_2tx_fpga/channel_estimator/peakdetect_ch2/correlator2/rx_ram_q_instance56/get_bit/get_bit ==
  data: u input; y output; ind input
function y = fcn(u,ind)
%#codegen

y = logical(bitget(u,ind));

== matlab function gm_ZynqBF_2tx_fpga/channel_estimator/peakdetect_ch2/correlator2/rx_ram_q_instance57/get_bit/get_bit ==
  data: u input; y output; ind input
function y = fcn(u,ind)
%#codegen

y = logical(bitget(u,ind));

== matlab function gm_ZynqBF_2tx_fpga/channel_estimator/peakdetect_ch2/correlator2/rx_ram_q_instance58/get_bit/get_bit ==
  data: u input; y output; ind input
function y = fcn(u,ind)
%#codegen

y = logical(bitget(u,ind));

== matlab function gm_ZynqBF_2tx_fpga/channel_estimator/peakdetect_ch2/correlator2/rx_ram_q_instance59/get_bit/get_bit ==
  data: u input; y output; ind input
function y = fcn(u,ind)
%#codegen

y = logical(bitget(u,ind));

== matlab function gm_ZynqBF_2tx_fpga/channel_estimator/peakdetect_ch2/correlator2/rx_ram_q_instance60/get_bit/get_bit ==
  data: u input; y output; ind input
function y = fcn(u,ind)
%#codegen

y = logical(bitget(u,ind));

== matlab function gm_ZynqBF_2tx_fpga/channel_estimator/peakdetect_ch2/correlator2/rx_ram_q_instance61/get_bit/get_bit ==
  data: u input; y output; ind input
function y = fcn(u,ind)
%#codegen

y = logical(bitget(u,ind));

== matlab function gm_ZynqBF_2tx_fpga/channel_estimator/peakdetect_ch2/correlator2/rx_ram_q_instance62/get_bit/get_bit ==
  data: u input; y output; ind input
function y = fcn(u,ind)
%#codegen

y = logical(bitget(u,ind));

== matlab function gm_ZynqBF_2tx_fpga/channel_estimator/peakdetect_ch2/correlator2/rx_ram_q_instance63/get_bit/get_bit ==
  data: u input; y output; ind input
function y = fcn(u,ind)
%#codegen

y = logical(bitget(u,ind));

== matlab function gm_ZynqBF_2tx_fpga/channel_estimator/peakdetect_ch2/correlator2/rx_ram_q_instance64/get_bit/get_bit ==
  data: u input; y output; ind input
function y = fcn(u,ind)
%#codegen

y = logical(bitget(u,ind));

== matlab function gm_ZynqBF_2tx_fpga/channel_estimator/ch_est/select_inputs/select_inputs ==
  data: en1 input; y output; en2 input; in1 input; in2 input
function y = fcn(en1, en2, in1, in2)
%#codegen

if (en1 && en2)
    y = zeros(2,1,'like',in1);
elseif (en1)
    y = in1;
elseif (en2)
    y = in2;
else
    y = zeros(2,1,'like',in1);
end
